simulink model "TestSplitter"  (R2013b)
settings: Solver=ode45  StartTime=0.0  StopTime=10.0  RelTol=1e-3
libraries: Lib_TurboC_FlowStart_TMATSC x1, Lib_TurboC_Splitter_TMATSC x1
settings Model: Creator=tlavelle  LastModifiedBy=jwchapm2
settings OptimizationCC: ExpressionDepthLimit=2147483647
settings DebuggingCC: StateNameClashWarn=warning

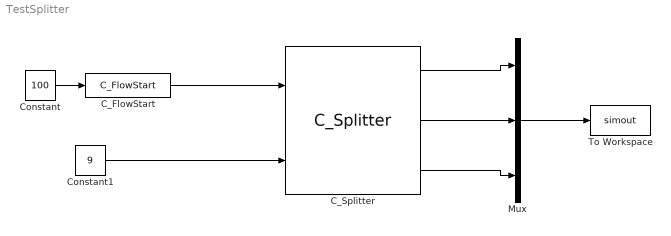
== system TestSplitter ==
  C_FlowStart : Lib_TurboC_FlowStart_TMATSC/C_FlowStart  Tt_M=500  Pt_M=15  comp1_M=1  comp2_M=0  comp3_M=0  comp4_M=0  comp5_M=0  comp6_M=0
  C_Splitter : Lib_TurboC_Splitter_TMATSC/C_Splitter
  Constant : Constant  Value=100
  Constant1 : Constant  Value=9
  Mux : Mux  Inputs=3
  To Workspace : ToWorkspace  VariableName=simout  SampleTime=-1  SaveFormat=Timeseries
  wires:
  Constant/1 -> C_FlowStart/1
  C_FlowStart/1 -> C_Splitter/1
  Constant1/1 -> C_Splitter/2
  C_Splitter/1 -> Mux/1
  C_Splitter/2 -> Mux/2
  Mux/1 -> To Workspace/1
  C_Splitter/3 -> Mux/3
